simulink model "ch_tan"  (R2015b)
settings: Solver=VariableStepAuto  StartTime=0.0  StopTime=10.0  RelTol=1e-3
libraries: simulink x1
settings Model: Creator=Chaohua Zhao  LastModifiedBy=Chaohua Zhao

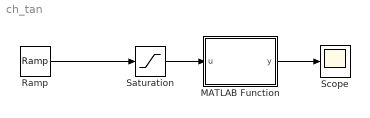
== system ch_tan ==
  MATLAB Function : MATLAB Function  TreatAsAtomicUnit=on
  Ramp : simulink/Sources/Ramp  slope=1  start=0  X0=0
  Saturation : Saturate  UpperLimit=2*pi  LowerLimit=0
  Scope : Scope
  wires:
  Ramp/1 -> Saturation/1
  Saturation/1 -> MATLAB Function/1(u)
  MATLAB Function/1(y) -> Scope/1

== matlab function ch_tan/MATLAB Function ==
  data: u input; y output
function y = fcn(u)
%#codegen

y = tan(u);
